simulink model "e5090s21pFinal_simulink_REV2"  (R2020b)
settings: Solver=VariableStepAuto  StartTime=0.0  StopTime=30  RelTol=1e-3
undefined symbols (not defined in the file): Dz_PIDF, gainBlock, regstatevarz, tfden, tfnum, Ts
libraries: dspsigops x1
settings Model: Creator=Rafael.Medeiros  LastModifiedBy=Rafael.Medeiros
settings SolverCC: AlgebraicLoopSolver=LineSearch

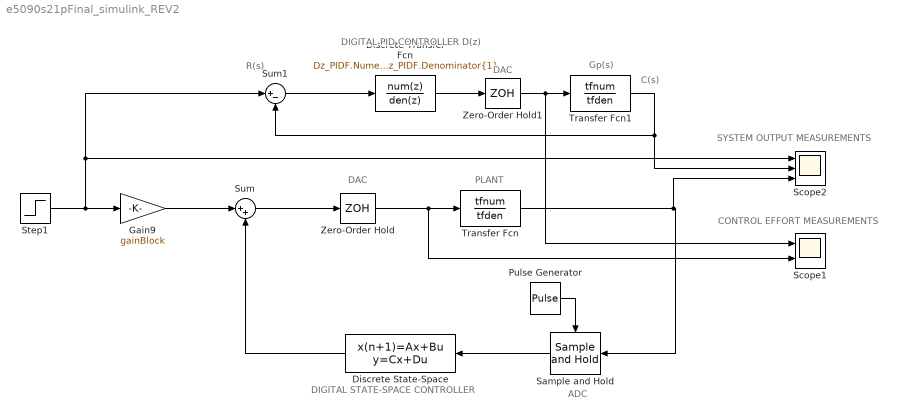
== system e5090s21pFinal_simulink_REV2 ==
  note: C(s)
  note: R(s)
  note: CONTROL EFFORT MEASUREMENTS
  note: SYSTEM OUTPUT MEASUREMENTS
  note: Gp(s)
  note: DAC
  note: DIGITAL PID CONTROLLER
      | D(z)
  note: DIGITAL STATE-SPACE CONTROLLER
  note: ADC
  note: PLANT
  note: DAC
  Discrete Transfer Fcn : DiscreteTransferFcn  Numerator=Dz_PIDF.Numerator{1}  Denominator=Dz_PIDF.Denominator{1}
  Discrete State-Space : DiscreteStateSpace  A=regstatevarz.A  B=regstatevarz.B  C=regstatevarz.C  D=regstatevarz.D  SampleTime=-1
  Gain9 : Gain  Gain=gainBlock
  Pulse Generator : DiscretePulseGenerator  PulseType=Time based  Period=Ts  PulseWidth=5
  Sample and Hold : dspsigops/Sample and Hold  trig=Rising edge  initCond=0  latchinput=off
  Scope1 : Scope  NumInputPorts=2
  Scope2 : Scope  NumInputPorts=3
  Step1 : Step  Time=0  SampleTime=0
  Sum : Sum  Inputs=|++
  Sum1 : Sum  Inputs=|+-
  Transfer Fcn : TransferFcn  Numerator=tfnum  Denominator=tfden
  Transfer Fcn1 : TransferFcn  Numerator=tfnum  Denominator=tfden
  Zero-Order Hold : ZeroOrderHold  SampleTime=Ts
  Zero-Order Hold1 : ZeroOrderHold  SampleTime=Ts
  wires:
  Step1/1 -> Sum1/1, Scope2/1, Gain9/1
  Zero-Order Hold/1 -> Scope1/2, Transfer Fcn/1
  Pulse Generator/1 -> Sample and Hold/Trigger
  Discrete State-Space/1 -> Sum/2
  Gain9/1 -> Sum/1
  Sum/1 -> Zero-Order Hold/1
  Sample and Hold/1 -> Discrete State-Space/1
  Transfer Fcn/1 -> Scope2/3, Sample and Hold/1
  Discrete Transfer Fcn/1 -> Zero-Order Hold1/1
  Zero-Order Hold1/1 -> Scope1/1, Transfer Fcn1/1
  Sum1/1 -> Discrete Transfer Fcn/1
  Transfer Fcn1/1 -> Scope2/2, Sum1/2
